simulink model "Tau_Observer_for_non_linear_system"  (R2017a)
settings: Solver=VariableStepAuto  StartTime=0.0  StopTime=2  RelTol=1e-3
values from neighbouring files (symbols this model uses):
  A = [0 1;0 0]    [Adaptive_Control.m]    (also in Adaptive_Control_Linear.m = [0 1;a1 a2]; HGO.m = [0 1;-1 -1]; Non_linear_observers_.m; feedback-integrator.m = [1 1;0 0])
  L = [3 1]'    [Non_linear_observers_.m]    (also in projet_AAV.m = 1; testing_linear_observer.m = L')
settings Model: Creator=firass2019  LastModifiedBy=firass2019

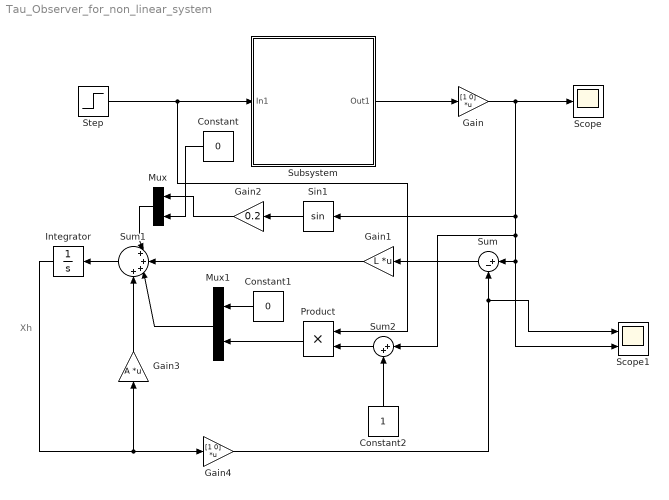
== system Tau_Observer_for_non_linear_system ==
  note: Xh
  Constant : Constant  Value=0
  Constant1 : Constant  Value=0
  Constant2 : Constant
  Gain : Gain  Gain=[1 0]  Multiplication=Matrix(K*u)
  Gain1 : Gain  Gain=L  Multiplication=Matrix(K*u)
  Gain2 : Gain  Gain=0.2
  Gain3 : Gain  Gain=A  Multiplication=Matrix(K*u)
  Gain4 : Gain  Gain=[1 0]  Multiplication=Matrix(K*u)
  Integrator : Integrator
  Mux : Mux  Inputs=2
  Mux1 : Mux  Inputs=2
  Product : Product
  Scope : Scope
  Scope1 : Scope  NumInputPorts=2
  Sin1 : Trigonometry
  Step : Step  SampleTime=0
  Subsystem : Subsystem
  Sum : Sum  Inputs=|+-
  Sum1 : Sum  Inputs=|++++
  Sum2 : Sum  Inputs=|++
  wires:
  Step/1 -> Product/1, Subsystem/1(In1)
  Subsystem/1(Out1) -> Gain/1
  Gain/1 -> Sin1/1, Sum2/1, Scope1/2, Sum/1, Scope/1
  Sum/1 -> Gain1/1
  Gain4/1 -> Scope1/1, Sum/2
  Sin1/1 -> Gain2/1
  Constant/1 -> Mux/2
  Gain2/1 -> Mux/1
  Mux/1 -> Sum1/1
  Gain3/1 -> Sum1/4
  Constant1/1 -> Mux1/1
  Constant2/1 -> Sum2/2
  Sum2/1 -> Product/2
  Product/1 -> Mux1/2
  Sum1/1 -> Integrator/1
  Integrator/1 -> Gain3/1, Gain4/1
  Mux1/1 -> Sum1/3
  Gain1/1 -> Sum1/2

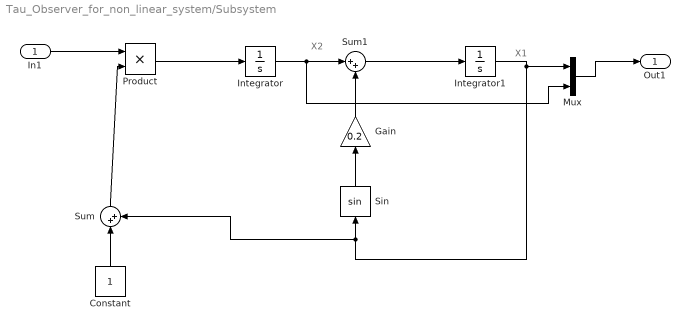
== system Tau_Observer_for_non_linear_system/Subsystem ==
  note: X2
  note: X1
  In1 : Inport
  Constant : Constant
  Gain : Gain  Gain=0.2
  Integrator : Integrator
  Integrator1 : Integrator  InitialCondition=0.5
  Mux : Mux  Inputs=2
  Product : Product
  Sin : Trigonometry
  Sum : Sum  Inputs=|++
  Sum1 : Sum  Inputs=|++
  Out1 : Outport
  wires:
  Sin/1 -> Gain/1
  Sum1/1 -> Integrator1/1
  Integrator1/1 -> Mux/1, Sum/2, Sin/1
  Mux/1 -> Out1/1
  Sum/1 -> Product/2
  In1/1 -> Product/1
  Constant/1 -> Sum/1
  Product/1 -> Integrator/1
  Gain/1 -> Sum1/2
  Integrator/1 -> Mux/2, Sum1/1
